simulink library "Brakes_Elements"  (R2026a)
settings: Solver=VariableStepAuto
undefined symbols (not defined in the file): brk_filt_fa, brk_max_p_fa, valve_leak, valve_maxA, valve_maxO, valve_ts, valve_x0
libraries: fl_lib x6, nesl_utility x2, sh_lib x2, Custom_lib x1
Description:
  | Component of Simscape Vehicle Templates Library
  | 
  | Copyright 2018-2026 The MathWorks, Inc.
settings Model: Creator=smiller  LastModifiedBy=smiller

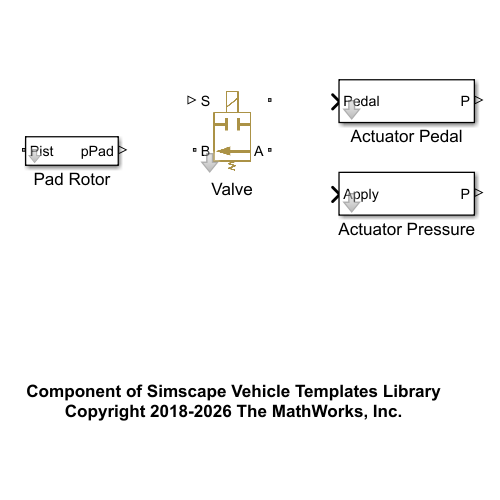
[thumbnail: Simulink's stored preview of the top-level diagram]
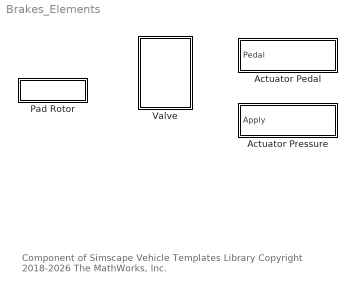
== system Brakes_Elements ==
  note: Component of Simscape Vehicle Templates Library
      | Copyright 2018-2026 The MathWorks, Inc.
  Actuator Pedal : Subsystem  mask(Brake Actuator, Pedal Input){brk_max_p=brk_max_p_fa, brk_filt=brk_filt_fa}
      mask prompts: brk_max_p "Max Pad Pressure (Pa)"; brk_filt "Time Constant (s)"
      mask help: Models brake actuator dynamics. A transfer function models delay from brake pedal movement to pressure applied at brake rotor.
      mask TypeOptions brk_max_p: Filter/Numerator
  Actuator Pressure : Subsystem  mask(Brake Actuator, Pressure Input){brk_filt=brk_filt_fa}
      mask prompts: brk_filt "Time Constant (s)"
      mask help: Models brake actuator dynamics. A transfer function models delay from pressure request from the control system to applying pressure at brake rotor.
  Pad Rotor : Subsystem  mask(Pad Rotor Contact){d_caliper_piston_f=0.01}
      mask prompts: d_caliper_piston_f "Front Caliper Piston Bore (m)"
      mask help: Models contact between pad and rotor. Determines pressure applied at rotor.
      mask TypeOptions d_caliper_piston_f:
      | Rotor Force
      | to Pad Pressure/cylinder_bore
  Valve : Subsystem  mask(Custom Two-Way Faultable Valve){area_max=valve_maxA, opening_max=valve_maxO, A_leak=valve_leak, x_0=valve_x0, time_constant=valve_ts, popup_openClose=Open, popup_fault=None}
      mask prompts: area_max "Valve passage maximum area"; opening_max "Valve maximum opening"; A_leak "Leakage area"; x_0 "Initial opening"; time_constant "Time constant"; popup_openClose "Nominally Open/Closed (image)"; popup_fault "Fault"
      mask help: Model two-way valve with optional degraded behavior.
      mask init:
      | if(strcmp(get_param(gcb,'popup_fault'),'None')) 
      |     set_param(gcb,'BackGroundColor','[1 1 1]');
      | else
      |     set_param(gcb,'BackGroundColor','[1.0, 0.85, 0.85]')
      | end
      mask TypeOptions area_max: Valve/area_max
      mask TypeOptions opening_max: Valve/opening_max | Valve Actuator/valve_stroke
      mask TypeOptions A_leak: Valve/A_leak
      mask TypeOptions x_0: Valve/x_0
      mask TypeOptions time_constant: Valve Actuator/time_constant
      mask TypeOptions popup_openClose: Open | Closed
      mask TypeOptions popup_fault: None | Stuck Open | Stuck Closed | Partial Open | Partial Close
      mask DialogControl Container4 Prompt: Geometry
      mask DialogControl Container8 Prompt: Fault
      mask Display:
      | if(strcmp(get_param(gcb,'popup_openClose'),'Open'))
      |     image('sm_car_2wayValve_nomOpen_IMAGE.png');
      | elseif(strcmp(get_param(gcb,'popup_openClose'),'Closed'))
      |     image('sm_car_2wayValve_IMAGE.png');
      | end

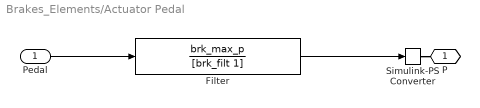
== system Brakes_Elements/Actuator Pedal ==
  Pedal : Inport
  Filter : TransferFcn  Numerator=brk_max_p  Denominator=[brk_filt 1]
  Simulink-PS Converter : nesl_utility/Simulink-PS Converter  PhysicalDomain=network_engine_domain  SubClassName=ps_input  LeftPortType=input  RightPortType=output  PseudoPeriodic=off  Frequencies=[]  NoiseDistribution=none  NoiseParameters=[]  Unit=1  AffineConversion=off  FilteringAndDerivatives=provide  SimscapeFilterOrder=1  InputFilterTimeConstant=0.001  UdotUserProvided=0
  P : PMIOPort  Side=Right
  wires:
  Pedal/1 -> Filter/1
  Filter/1 -> Simulink-PS Converter/1
  connections:
  Simulink-PS Converter/RConn1 -- P/RConn1

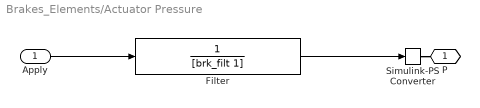
== system Brakes_Elements/Actuator Pressure ==
  Apply : Inport
  Filter : TransferFcn  Numerator=1  Denominator=[brk_filt 1]
  Simulink-PS Converter : nesl_utility/Simulink-PS Converter  PhysicalDomain=network_engine_domain  SubClassName=ps_input  LeftPortType=input  RightPortType=output  PseudoPeriodic=off  Frequencies=[]  NoiseDistribution=none  NoiseParameters=[]  Unit=1  AffineConversion=off  FilteringAndDerivatives=provide  SimscapeFilterOrder=1  InputFilterTimeConstant=0.001  UdotUserProvided=0
  P : PMIOPort  Side=Right
  wires:
  Filter/1 -> Simulink-PS Converter/1
  Apply/1 -> Filter/1
  connections:
  Simulink-PS Converter/RConn1 -- P/RConn1

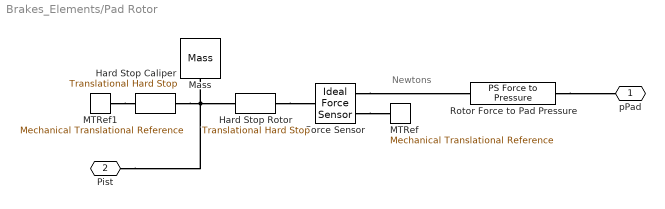
== system Brakes_Elements/Pad Rotor ==
  note: Newtons
  Force Sensor : fl_lib/Mechanical/Mechanical Sensors/Ideal Force Sensor
  Hard Stop Caliper : fl_lib/Mechanical/Translational Elements/Translational Hard Stop  upper_bnd=0.1 m  lower_bnd=0 m  model=1  stiff_up=1e6 N/m  stiff_low=1e6 N/m  D_up=150 N/(m/s)  D_low=150 N/(m/s)  transition=0.1 mm  coeff_rest=0.7  v_tol=0.001 m/s  f_tol=0.001 N  v_specify=off  v_priority=None  v=0 m/s  v_nominal_specify=off  v_nominal_value=1  v_nominal_unit=m/s  f_specify=off  f_priority=None  f=0 N  f_nominal_specify=off  f_nominal_value=1  f_nominal_unit=N  x_specify=off  x_priority=High  x=0 m  x_nominal_specify=off  x_nominal_value=1  x_nominal_unit=m  M_specify=off  M_priority=None  M=0
  Hard Stop Rotor : fl_lib/Mechanical/Translational Elements/Translational Hard Stop  upper_bnd=0.45*1e-3 m  lower_bnd=-0.1 m  model=1  stiff_up=1e9*1e-3 N/m  stiff_low=1e9*1e-3 N/m  D_up=1e6*1e-3 N/(m/s)  D_low=1e6*1e-3 N/(m/s)  transition=0.045*1e-3 m  coeff_rest=0.7  v_tol=0.001 m/s  f_tol=0.001 N  v_specify=off  v_priority=None  v=0 m/s  v_nominal_specify=off  v_nominal_value=1  v_nominal_unit=m/s  f_specify=off  f_priority=None  f=0 N  f_nominal_specify=off  f_nominal_value=1  f_nominal_unit=N  x_specify=off  x_priority=High  x=0 m  x_nominal_specify=off  x_nominal_value=1  x_nominal_unit=m  M_specify=off  M_priority=None  M=0
  MTRef : fl_lib/Mechanical/Translational Elements/Mechanical Translational Reference
  MTRef1 : fl_lib/Mechanical/Translational Elements/Mechanical Translational Reference
  Mass : fl_lib/Mechanical/Translational Elements/Mass  mass=0.3 kg  num_ports=foundation.enum.numPorts2.one  v_specify=off  v_priority=High  v=0 m/s  v_nominal_specify=off  v_nominal_value=1  v_nominal_unit=m/s  f_specify=off  f_priority=None  f=0 N  f_nominal_specify=off  f_nominal_value=1  f_nominal_unit=N
  Rotor Force to Pad Pressure : Custom_lib/PS Force to Pressure  cylinder_bore=d_caliper_piston_f m
  pPad : PMIOPort  Side=Left
  Pist : PMIOPort  Port=2  Side=Right
  connections:
  Rotor Force to Pad Pressure/RConn1 -- pPad/RConn1
  Hard Stop Rotor/RConn1 -- Force Sensor/LConn1
  Force Sensor/RConn1 -- MTRef/LConn1
  Pist/RConn1 -- Hard Stop Caliper/LConn1 -- Mass/LConn1 -- Hard Stop Rotor/LConn1
  MTRef1/LConn1 -- Hard Stop Caliper/RConn1
  Force Sensor/RConn2 -- Rotor Force to Pad Pressure/LConn1

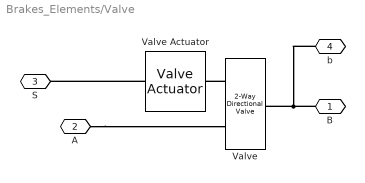
== system Brakes_Elements/Valve ==
  Valve : sh_lib/Valves/Directional Valves/2-Way Directional Valve  mdl_type=1  area_max=area_max mm^2  opening_max=opening_max m  opening_tab="[  -0.002 0 0.002 0.005 0.015 ] m"  area_tab="[  1e-09 2.0352e-07 4.0736e-05 0.00011438 0.00034356 ] m^2"  pressure_tab="[  -1e+07 -5e+06 -2e+06 2e+06 5e+06 1e+07 ] Pa"  flow_rate_tab="[  -1e-07 -7.0711e-08 -4.4721e-08 4.4721e-08 7.0711e-08 1e-07 ; -2.0352e-05 -1.4391e-05 -9.1017e-06 9.1017e-06 1.4391e-05 2.0352e-05 ; -0.0040736 -0.0028805 -0.0018218 0.0018218 0.0028805 0.0040736 ; -0.011438 -0.0080879 -0.0051152 0.0051152 0.0080879 0.011438 ; -0.034356 -0.024293 -0.015364 0.015364 0.024293 0.034356 ; ] m^3/s"  interp_method=1  extrap_method=1  C_d=0.7  x_0=x_0 m  A_leak=A_leak mm^2  lam_spec=2  B_lam=0.999  Re_cr=12
  Valve Actuator : sh_lib/Valves/Valve Actuators/Valve Actuator  valve_stroke=opening_max m  time_constant=time_constant s  gain=1 m
  B : PMIOPort  Side=Right
  A : PMIOPort  Port=2  Side=Left
  S : PMIOPort  Port=3  Side=Right
  b : PMIOPort  Port=4  Side=Left
  connections:
  A/RConn1 -- Valve/LConn2
  B/RConn1 -- b/RConn1 -- Valve/RConn1
  Valve Actuator/LConn1 -- S/RConn1
  Valve/LConn1 -- Valve Actuator/RConn1
